simulink model "Amp_baseline_Excel"  (R2020a)
settings: Solver=VariableStepAuto  StartTime=0.0  StopTime=60  RelTol=1e-3
model workspace (MAT data in the model file):
  WinSize = Simulink.Parameter
  WinSize.Value = 16
  WinSize.DataType = 'double'
  WinSize.Dimensions = [1 1]
  fc_bandpass = Simulink.Parameter
  fc_bandpass.Value = [0.05 0.26]
  fc_bandpass.DataType = 'double'
  fc_bandpass.Dimensions = [1 2]
undefined symbols (not defined in the file or in its folder): A1, A138674, A91496, C1, I1, J138674, O91496
settings Model: Creator=LAB-OREN3  LastModifiedBy=LAB-OREN3

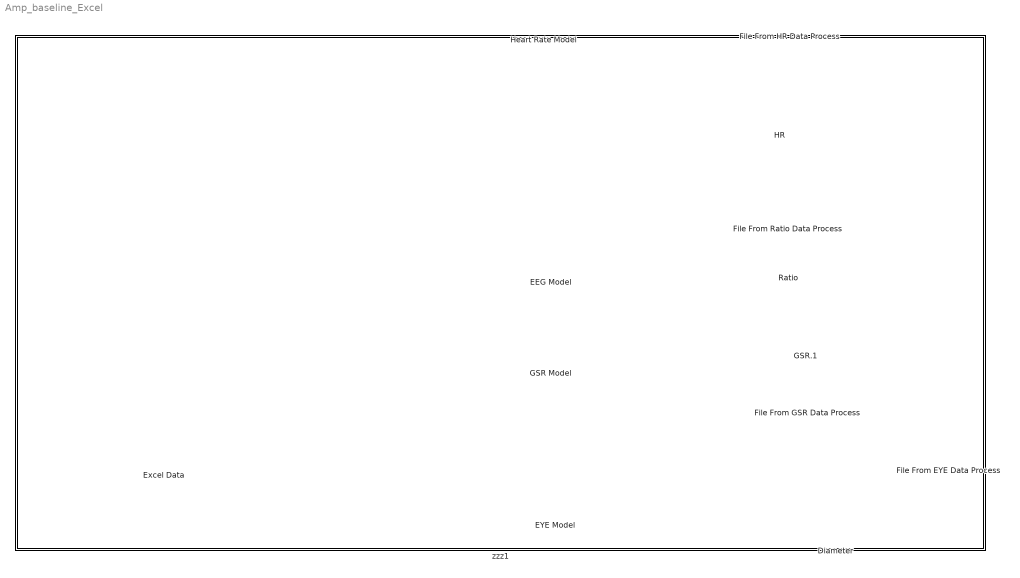
== system Amp_baseline_Excel ==
  Diameter : Display
  EEG Model : Subsystem  ReferencedSubsystem=EEG_Ratio_Model
  EYE Model : Subsystem  ReferencedSubsystem=Pupil_Diameter_Model_BaseLine
  Excel Data : Subsystem
  File From EYE Data Process : ToFile  Filename=Eye_Diameter.mat  MatrixName=Eye_Diameter
  File From GSR Data Process : ToFile  Filename=GSR.mat  MatrixName=GSR
  File From HR Data Process : ToFile  Filename=Heartrate_Test.mat  MatrixName=heartRatedata
  File From Ratio Data Process : ToFile  Filename=Ratio.mat  MatrixName=Ratio
  GSR Model : Subsystem
  GSR.1 : Display
  HR : Display
  Heart Rate Model : Subsystem  ReferencedSubsystem=Heart_Rate_Model
  Ratio : Display
  zzz1 : Subsystem  TreatAsAtomicUnit=on
      settings: OpenFcn=% no-op
      mask Display: disp('')
  wires:
  Heart Rate Model/1 -> File From HR Data Process/1
  GSR Model/1(GSR) -> File From GSR Data Process/1, GSR.1/1
  Heart Rate Model/2 -> HR/1
  EYE Model/1 -> File From EYE Data Process/1, Diameter/1
  EEG Model/1 -> Ratio/1, File From Ratio Data Process/1
  Excel Data/1(Out1) -> Heart Rate Model/1
  Excel Data/2(Out2) -> EEG Model/1
  Excel Data/3(Out3) -> EEG Model/2
  Excel Data/4(Out4) -> EEG Model/3
  Excel Data/5(Out5) -> EEG Model/4
  Excel Data/6(Out6) -> EEG Model/5
  Excel Data/7(Out7) -> EEG Model/6
  Excel Data/8(Out8) -> EEG Model/7
  Excel Data/9(Out9) -> EEG Model/8
  Excel Data/10(Out10) -> EEG Model/9
  Excel Data/11(Out11) -> EEG Model/10
  Excel Data/12(Out12) -> EEG Model/11
  Excel Data/13(Out13) -> GSR Model/1(In1)
  Excel Data/14(Out14) -> EYE Model/1
  Excel Data/15(Out15) -> EYE Model/2

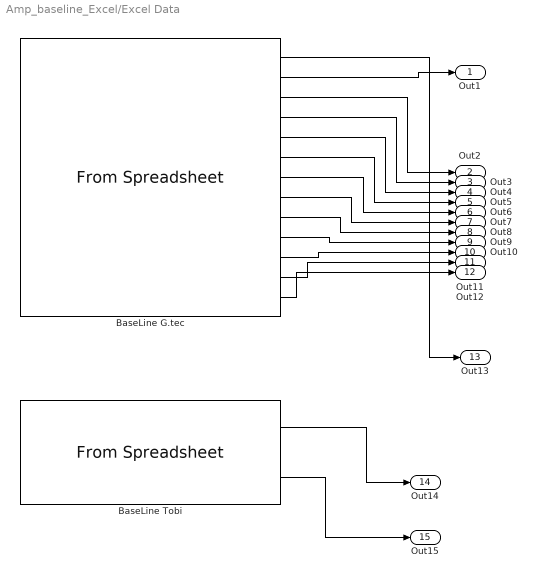
== system Amp_baseline_Excel/Excel Data ==
  BaseLine G.tec : FromSpreadsheet  FileName=C:\Users\LAB-OREN3\Downloads\1\g.techAmp Data of A2_535986_COMBINED_CUBE_DELAY_50_TTC_15 at (15;28;36).xlsx  SheetName=גיליון1  Range=A1:A91496,C1:O91496  SampleTime=0.001953125
  BaseLine Tobi : FromSpreadsheet  FileName=C:\Users\LAB-OREN3\Desktop\CognataData\Participants_DATA\Test\4\Tobii Data of A1_546053_TRAINING at (12;02;18).xlsx  SheetName=גיליון1  Range=A1:A138674,I1:J138674  SampleTime=0.001953125
  Out1 : Outport
  Out2 : Outport  Port=2
  Out3 : Outport  Port=3
  Out4 : Outport  Port=4
  Out5 : Outport  Port=5
  Out6 : Outport  Port=6
  Out7 : Outport  Port=7
  Out8 : Outport  Port=8
  Out9 : Outport  Port=9
  Out10 : Outport  Port=10
  Out11 : Outport  Port=11
  Out12 : Outport  Port=12
  Out13 : Outport  Port=13
  Out14 : Outport  Port=14
  Out15 : Outport  Port=15
  wires:
  BaseLine G.tec/2 -> Out1/1
  BaseLine G.tec/8 -> Out7/1
  BaseLine G.tec/13 -> Out12/1
  BaseLine Tobi/1 -> Out14/1
  BaseLine G.tec/4 -> Out3/1
  BaseLine G.tec/10 -> Out9/1
  BaseLine G.tec/6 -> Out5/1
  BaseLine G.tec/12 -> Out11/1
  BaseLine G.tec/3 -> Out2/1
  BaseLine G.tec/11 -> Out10/1
  BaseLine G.tec/9 -> Out8/1
  BaseLine G.tec/7 -> Out6/1
  BaseLine G.tec/5 -> Out4/1
  BaseLine Tobi/2 -> Out15/1
  BaseLine G.tec/1 -> Out13/1

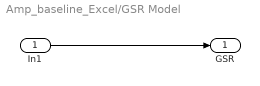
== system Amp_baseline_Excel/GSR Model ==
  In1 : Inport
  GSR : Outport
  wires:
  In1/1 -> GSR/1

== system Amp_baseline_Excel/zzz1 ==
